simulink model "A_sim"  (R2019b)
settings: Solver=VariableStepAuto  StartTime=0.0  StopTime=0.4  RelTol=1e-3
libraries: simulink_extras x2
settings Model: Creator=Shishir  LastModifiedBy=Shishir

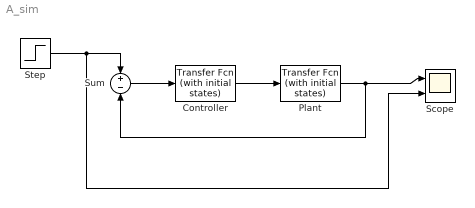
== system A_sim ==
  Controller : simulink_extras/Additional Linear/Transfer Fcn (with initial states)  N=[113.34]  D=[1 67.1]  X0=0
  Plant : simulink_extras/Additional Linear/Transfer Fcn (with initial states)  N=[100]  D="[1  25]"  X0=0
  Scope : Scope  NumInputPorts=2
  Step : Step  Time=0  SampleTime=0
  Sum : Sum  Inputs=+-
  wires:
  Controller/1 -> Plant/1
  Plant/1 -> Sum/2, Scope/1
  Sum/1 -> Controller/1
  Step/1 -> Sum/1, Scope/2
